simulink model "emg_live_simulink"  (R2025b)
settings: Solver=FixedStepDiscrete  StartTime=0.0  StopTime=inf  FixedStep=0.002  RelTol=1e-3
settings Model: Creator=ADMIN  LastModifiedBy=ADMIN

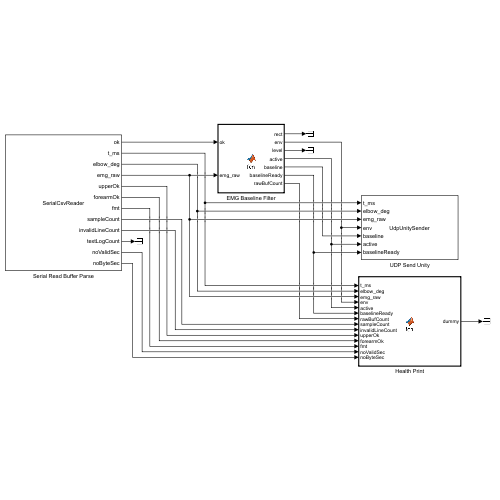
[thumbnail: Simulink's stored preview of the top-level diagram]
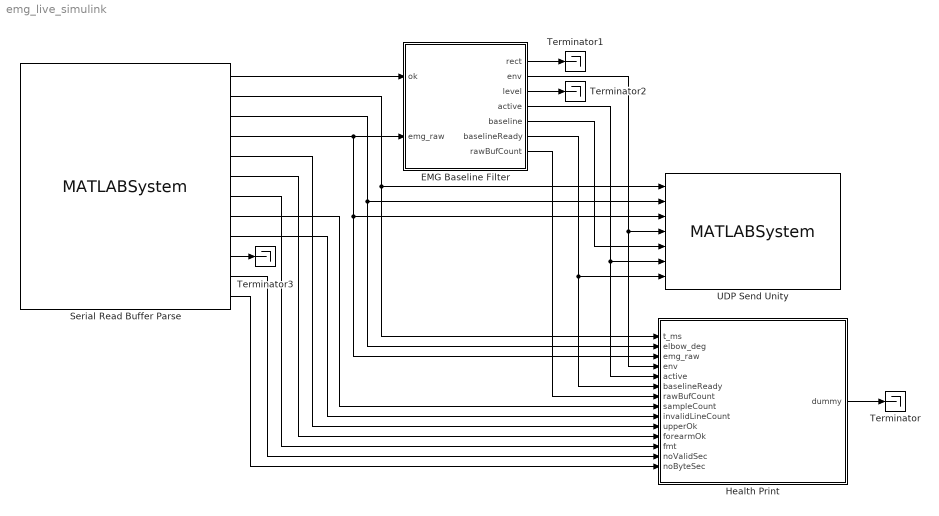
== system emg_live_simulink ==
  EMG Baseline Filter : MATLAB Function  TreatAsAtomicUnit=on
  Health Print : MATLAB Function  TreatAsAtomicUnit=on
  Serial Read Buffer Parse : MATLABSystem  System=SerialCsvReader  PORT=COM9  BAUD=115200  Timeout=0.02
      mask Type: SerialCsvReader
  Terminator{,1..3} (4 alike) : Terminator
  UDP Send Unity : MATLABSystem  System=UdpUnitySender  UNITY_IP=127.0.0.1  UNITY_PORT=55001  SEND_TO_UNITY=true  UDP_RATE_HZ=30
      mask Type: UdpUnitySender
  wires:
  Serial Read Buffer Parse/1 -> EMG Baseline Filter/1(ok)
  Serial Read Buffer Parse/4 -> UDP Send Unity/3, Health Print/3(emg_raw), EMG Baseline Filter/2(emg_raw)
  Serial Read Buffer Parse/2 -> Health Print/1(t_ms), UDP Send Unity/1
  Serial Read Buffer Parse/3 -> Health Print/2(elbow_deg), UDP Send Unity/2
  EMG Baseline Filter/2(env) -> Health Print/4(env), UDP Send Unity/4
  EMG Baseline Filter/5(baseline) -> UDP Send Unity/5
  EMG Baseline Filter/4(active) -> Health Print/5(active), UDP Send Unity/6
  EMG Baseline Filter/6(baselineReady) -> Health Print/6(baselineReady), UDP Send Unity/7
  EMG Baseline Filter/7(rawBufCount) -> Health Print/7(rawBufCount)
  Serial Read Buffer Parse/8 -> Health Print/8(sampleCount)
  Serial Read Buffer Parse/9 -> Health Print/9(invalidLineCount)
  Serial Read Buffer Parse/5 -> Health Print/10(upperOk)
  Serial Read Buffer Parse/6 -> Health Print/11(forearmOk)
  Serial Read Buffer Parse/7 -> Health Print/12(fmt)
  Serial Read Buffer Parse/11 -> Health Print/13(noValidSec)
  Serial Read Buffer Parse/12 -> Health Print/14(noByteSec)
  Health Print/1(dummy) -> Terminator/1
  Serial Read Buffer Parse/10 -> Terminator3/1
  EMG Baseline Filter/1(rect) -> Terminator1/1
  EMG Baseline Filter/3(level) -> Terminator2/1

== matlab function emg_live_simulink/Health Print ==
  data: t_ms input; dummy output; elbow_deg input; emg_raw input; env input; active input; baselineReady input; rawBufCount input; sampleCount input; invalidLineCount input; upperOk input; forearmOk input; fmt input; noValidSec input; noByteSec input
function dummy = fcn(t_ms, elbow_deg, emg_raw, env, active, ...
    baselineReady, rawBufCount, sampleCount, invalidLineCount, ...
    upperOk, forearmOk, fmt, noValidSec, noByteSec)
% Health print giống printHealth trong run_emg_live_local.m

PRINT_RATE_HZ = 1;
minPrintPeriod = 1 / PRINT_RATE_HZ;

persistent lastPrint initialized

if isempty(initialized)
    lastPrint = tic;
    initialized = true;
end

dummy = 0;

if toc(lastPrint) < minPrintPeriod
    return;
end

if sampleCount == 0
    fprintf("[CHECK] Serial bytes seen %.1fs ago | valid samples = 0 | waiting Arduino/MPU/CSV...\n", ...
        noByteSec);
    lastPrint = tic;
    return;
end

% fmt:
% 1 = mpu_success_15col
% 2 = test_6col
% 3 = main_3col

if fmt == 1 || fmt == 2
    if upperOk == 1 && forearmOk == 1

        if ~baselineReady
            fprintf("[CHECK] MPU OK: 0x68=1, 0x69=1 | BASELINE %.0f/200 | UDP WAIT BASELINE | samples=%.0f | invalid=%.0f | t=%8.0f ms | elbow=%7.2f | raw=%4.0f | env=%7.2f | active=%.0f | noCSV=%.1fs\n", ...
                rawBufCount, sampleCount, invalidLineCount, t_ms, elbow_deg, emg_raw, env, double(active), noValidSec);
        else
            if emg_raw <= 2 || emg_raw >= 1021
                fprintf("[CHECK] MPU OK: 0x68=1, 0x69=1 | EMG WARNING: ADC near rail | UDP ON | samples=%.0f | invalid=%.0f | t=%8.0f ms | elbow=%7.2f | raw=%4.0f | env=%7.2f | active=%.0f | noCSV=%.1fs\n", ...
                    sampleCount, invalidLineCount, t_ms, elbow_deg, emg_raw, env, double(active), noValidSec);
            else
                fprintf("[CHECK] MPU OK: 0x68=1, 0x69=1 | EMG OK | UDP ON | samples=%.0f | invalid=%.0f | t=%8.0f ms | elbow=%7.2f | raw=%4.0f | env=%7.2f | active=%.0f | noCSV=%.1fs\n", ...
                    sampleCount, invalidLineCount, t_ms, elbow_deg, emg_raw, env, double(active), noValidSec);
            end
        end

    else

        if ~baselineReady
            fprintf("[CHECK] MPU WARNING: 0x68=%.0f, 0x69=%.0f | BASELINE %.0f/200 | UDP WAIT BASELINE | samples=%.0f | invalid=%.0f | t=%8.0f ms | elbow=%7.2f | raw=%4.0f | env=%7.2f | active=%.0f | noCSV=%.1fs\n", ...
                upperOk, forearmOk, rawBufCount, sampleCount, invalidLineCount, t_ms, elbow_deg, emg_raw, env, double(active), noValidSec);
        else
            if emg_raw <= 2 || emg_raw >= 1021
                fprintf("[CHECK] MPU WARNING: 0x68=%.0f, 0x69=%.0f | EMG WARNING: ADC near rail | UDP ON | samples=%.0f | invalid=%.0f | t=%8.0f ms | elbow=%7.2f | raw=%4.0f | env=%7.2f | active=%.0f | noCSV=%.1fs\n", ...
                    upperOk, forearmOk, sampleCount, invalidLineCount, t_ms, elbow_deg, emg_raw, env, double(active), noValidSec);
            else
                fprintf("[CHECK] MPU WARNING: 0x68=%.0f, 0x69=%.0f | EMG OK | UDP ON | samples=%.0f | invalid=%.0f | t=%8.0f ms | elbow=%7.2f | raw=%4.0f | env=%7.2f | active=%.0f | noCSV=%.1fs\n", ...
                    upperOk, forearmOk, sampleCount, invalidLineCount, t_ms, elbow_deg, emg_raw, env, double(active), noValidSec);
            end
        end

    end

else
    if ~baselineReady
        fprintf("[CHECK] MPU DATA OK | BASELINE %.0f/200 | UDP WAIT BASELINE | samples=%.0f | invalid=%.0f | t=%8.0f ms | elbow=%7.2f | raw=%4.0f | env=%7.2f | active=%.0f | noCSV=%.1fs\n", ...
            rawBufCount, sampleCount, invalidLineCount, t_ms, elbow_deg, emg_raw, env, double(active), noValidSec);
    else
        if emg_raw <= 2 || emg_raw >= 1021
            fprintf("[CHECK] MPU DATA OK | EMG WARNING: ADC near rail | UDP ON | samples=%.0f | invalid=%.0f | t=%8.0f ms | elbow=%7.2f | raw=%4.0f | env=%7.2f | active=%.0f | noCSV=%.1fs\n", ...
                sampleCount, invalidLineCount, t_ms, elbow_deg, emg_raw, env, double(active), noValidSec);
        else
            fprintf("[CHECK] MPU DATA OK | EMG OK | UDP ON | samples=%.0f | invalid=%.0f | t=%8.0f ms | elbow=%7.2f | raw=%4.0f | env=%7.2f | active=%.0f | noCSV=%.1fs\n", ...
                sampleCount, invalidLineCount, t_ms, elbow_deg, emg_raw, env, double(active), noValidSec);
        end
    end
end

lastPrint = tic;
end

== matlab function emg_live_simulink/EMG Baseline Filter ==
  data: ok input; rect output; emg_raw input; env output; level output; active output; baseline output; baselineReady output; rawBufCount output
function [rect, env, level, active, baseline, baselineReady, rawBufCount] = fcn(ok, emg_raw)
% EMG Baseline + Butterworth filter
% Giữ đúng thuật toán từ run_emg_live_local.m
%
% fs = 100 Hz
% N  = 2
% fc = 5 Hz
% [b,a] = butter(2, 5/(100/2), "low")

BASELINE_SAMPLES = 200;
THRESHOLD_DELTA = 35;
LEVEL_SCALE = 512.0;

% Butterworth low-pass order 2, fc = 5 Hz, fs = 100 Hz
b0 = 0.020083365564211;
b1 = 0.040166731128423;
b2 = 0.020083365564211;

a1 = -1.561018075800718;
a2 = 0.641351538057563;

persistent rawBuf count baseline_p z1 z2 initialized

if isempty(initialized)
    rawBuf = zeros(1, BASELINE_SAMPLES);
    count = 0;
    baseline_p = NaN;

    % Direct Form II Transposed filter states
    z1 = 0;
    z2 = 0;

    initialized = true;
end

rect = 0;
env = 0;
level = 0;
active = false;
baseline = baseline_p;
baselineReady = ~isnan(baseline_p);
rawBufCount = count;

if ~ok
    return;
end

if isnan(baseline_p)
    count = count + 1;

    if count <= BASELINE_SAMPLES
        rawBuf(count) = emg_raw;
    else
        rawBuf(BASELINE_SAMPLES) = emg_raw;
    end

    tempBaseline = median(rawBuf(1:count));

    rect = abs(emg_raw - tempBaseline);
    env = 0;
    level = 0;
    active = false;

    if count >= BASELINE_SAMPLES
        baseline_p = median(rawBuf(1:BASELINE_SAMPLES));

        fprintf("\n[OK] EMG baseline ready: %.2f ADC from %.0f samples.\n", baseline_p, count);
        fprintf("[RUN] Simulink is now sending elbow + filtered EMG to Unity.\n\n");
    end
else
    rect = abs(emg_raw - baseline_p);

    % Equivalent to:
    % [env, zi] = filter(b, a, rect, zi);
    env = b0 * rect + z1;
    z1_new = b1 * rect + z2 - a1 * env;
    z2_new = b2 * rect - a2 * env;
    z1 = z1_new;
    z2 = z2_new;

    level = min(max(env / LEVEL_SCALE, 0), 1);
    active = env > THRESHOLD_DELTA;
end

baseline = baseline_p;
baselineReady = ~isnan(baseline_p);
rawBufCount = count;
end
